simulink model "Ground_Vehicle_Model"  (R2020b)
settings: Solver=VariableStepAuto  StartTime=0.0  StopTime=40000  RelTol=1e-3
values from neighbouring files (symbols this model uses):
  waypoint = [waypoint(1,:);waypoint(1,:)]    [Path_Planning_Algorithm.m]
  Waypoint_Number = Waypoint_Number+1    [Path_Planning_Algorithm.m]
  waypoint_with_start = [0 0 0 0 0;waypoint]    [Path_Planning_Algorithm.m]
libraries: pid_lib x4, simulink x1, dspswit3 x1
settings Model: Creator=fuska  LastModifiedBy=fuska
settings DebuggingCC: AlgebraicLoopMsg=none

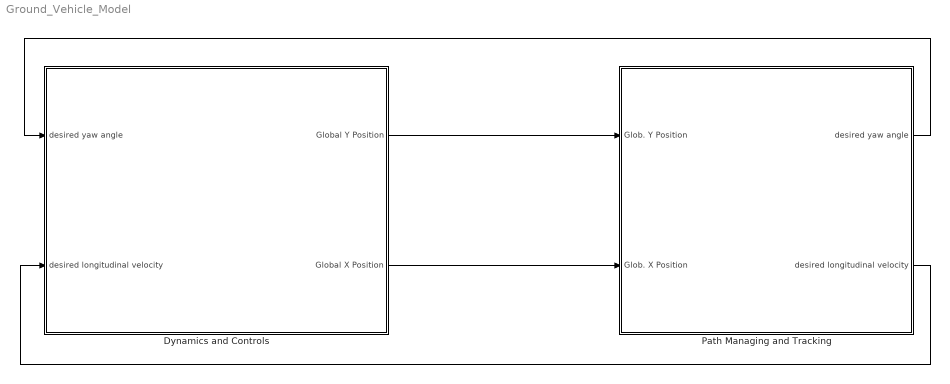
== system Ground_Vehicle_Model ==
  Dynamics and Controls : Subsystem
  Path Managing and Tracking : Subsystem
  wires:
  Dynamics and Controls/1(Global Y Position) -> Path Managing and Tracking/1(Glob. Y Position)
  Dynamics and Controls/2(Global X Position) -> Path Managing and Tracking/2(Glob. X Position)
  Path Managing and Tracking/1(desired yaw angle) -> Dynamics and Controls/1(desired yaw angle)
  Path Managing and Tracking/2(desired longitudinal velocity) -> Dynamics and Controls/2(desired longitudinal velocity)

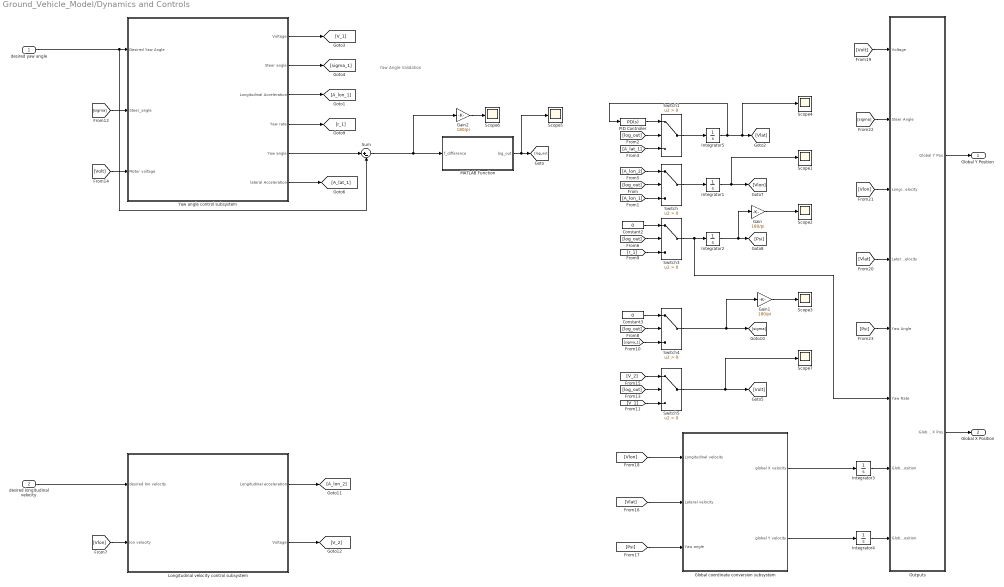
== system Ground_Vehicle_Model/Dynamics and Controls ==
  note: Yaw Angle Validation
  desired yaw angle : Inport
  desired longitudinal velocity : Inport  Port=2
  Constant2 : Constant  Value=0
  Constant3 : Constant  Value=0
  Gain : Gain  Gain=180/pi
  Gain1 : Gain  Gain=180/pi
  Gain2 : Gain  Gain=180/pi
  Global coordinate conversion subsystem : Subsystem
  Integrator{1..5} (5 alike) : Integrator
  Longitudinal velocity control subsystem : Subsystem
  MATLAB Function : MATLAB Function  TreatAsAtomicUnit=on
  Outputs : Subsystem
  PID Controller : pid_lib/PID Controller  Controller=PD  Form=Parallel  TimeDomain=Continuous-time  UseExternalTs=off  SampleTime=-1  IntegratorMethod=Forward Euler  FilterMethod=Forward Euler  ControllerParametersSource=internal  P=-0.8*9.81  I=1  D=0  UseFilter=on  N=100  TunerSelectOption=Transfer Function Based (PID Tuner App)  InitialConditionSource=internal  InitialConditionForIntegrator=0  InitialConditionForFilter=0  DifferentiatorICPrevScaledInput=0  ExternalReset=none  TrackingMode=off  Kt=1  LimitOutput=off  SatLimitsSource=internal  UpperSaturationLimit=inf  LowerSaturationLimit=-inf  LinearizeAsGain=on  AntiWindupMode=none  Kb=1  POutMin=[]  POutMax=[]  IOutMin=[]  IOutMax=[]  DOutMin=[]  DOutMax=[]  NOutMin=[]  NOutMax=[]  SumOutMin=[]  SumOutMax=[]  SaturationOutMin=[]  SaturationOutMax=[]  PParamMin=[]  PParamMax=[]  IParamMin=[]  IParamMax=[]  DParamMin=[]  DParamMax=[]  NParamMin=[]  NParamMax=[]  KbParamMin=[]  KbParamMax=[]  KtParamMin=[]  KtParamMax=[]  KbOutMin=[]  KbOutMax=[]  KtOutMin=[]  KtOutMax=[]  IntegratorOutMin=[]  IntegratorOutMax=[]  FilterOutMin=[]  FilterOutMax=[]  SumI1OutMin=[]  SumI1OutMax=[]  SumI2OutMin=[]  SumI2OutMax=[]  SumI3OutMin=[]  SumI3OutMax=[]  SumI4OutMin=[]  SumI4OutMax=[]  SumDOutMin=[]  SumDOutMax=[]  DifferentiatorOutMin=[]  DifferentiatorOutMax=[]  FilterDiffOutCoefMin=[]  FilterDiffOutCoefMax=[]  ReciprocalOutMin=[]  ReciprocalOutMax=[]  SumDenOutMin=[]  SumDenOutMax=[]  SumNumOutMin=[]  SumNumOutMax=[]  DivideOutMin=[]  DivideOutMax=[]  UdiffTsProdOutMin=[]  UdiffTsProdOutMax=[]  NTsProdOutMin=[]  NTsProdOutMax=[]  UintegralTsProdOutMin=[]  UintegralTsProdOutMax=[]  UngainTsProdOutMin=[]  UngainTsProdOutMax=[]  IntegratorContinuousStateAttributes=''  IntegratorStateMustResolveToSignalObject=off  IntegratorRTWStateStorageClass=Auto  FilterContinuousStateAttributes=''  FilterStateMustResolveToSignalObject=off  FilterRTWStateStorageClass=Auto  ParallelPVariant=InternalParameters  IdealPVariant=Disabled  IVariant=Disabled  DVariant=InternalParameters  IntegratorVariant=Disabled  SatVariant=Disabled  AWVariant=Disabled  PCopyVariant=Disabled  TRVariant=Disabled  FdbkBlocksVariant=Forward  IdealPFdbkVariant=Disabled  SatFdbkVariant=Disabled  DerivativeFilterVariant=ContFilter  NVariant=InternalParameters  NCopyVariant=Disabled  FilterICVariant=InternalICsFilter  IntegratorICVariant=Disabled  ExternalResetVariant=Disabled  TRSumVariant=Passthrough  SumFdbkVariant=Disabled  SumVariant=Sum_PD  TsampFilterVariant=InternalTs  TsampNgainVariant=Passthrough  TsampIntegralVariant=Disabled_SignalSpec  ExternalSaturationOutDataTypeStr=Inherit: Same as second input
  Scope{1..7} (7 alike) : Scope
  Sum : Sum  Inputs=|+-
  Switch{,1,3..5} (5 alike) : Switch  Criteria=u2 > Threshold
  Yaw angle control subsystem : Subsystem
  Global Y Position : Outport
  Global X Position : Outport  Port=2
  wires:
  desired yaw angle/1 -> Yaw angle control subsystem/1(Desired Yaw Angle), Sum/2
  Yaw angle control subsystem/5(Yaw angle) -> Sum/1
  Sum/1 -> Gain2/1, MATLAB Function/1(f_difference)
  MATLAB Function/1(log_out) -> Scope5/1, [log_out]
  [log_out] -> Switch/2
  Yaw angle control subsystem/3(Longitudinal Acceleration) -> [A_lon_1]
  [A_lon_1] -> Switch/3
  [A_lon_2] -> Switch/1
  Yaw angle control subsystem/1(Voltage) -> [V_1]
  Yaw angle control subsystem/2(Steer angle) -> [sigma_1]
  Switch/1 -> Integrator1/1
  Integrator1/1 -> Scope1/1, [Vlon]
  Integrator2/1 -> Gain/1, [Psi]
  Switch3/1 -> Outputs/6(Yaw Rate), Integrator2/1
  [log_out] -> Switch3/2
  [r_1] -> Switch3/3
  Constant2/1 -> Switch3/1
  Yaw angle control subsystem/4(Yaw rate) -> [r_1]
  Constant3/1 -> Switch4/1
  [sigma_1] -> Switch4/3
  [log_out] -> Switch4/2
  Switch4/1 -> Gain1/1, [sigma]
  [log_out] -> Switch5/2
  [V_1] -> Switch5/3
  Switch5/1 -> Scope7/1, [Volt]
  desired longitudinal velocity/1 -> Longitudinal velocity control subsystem/1(desired lon velocity)
  [Vlon] -> Longitudinal velocity control subsystem/2(lon velocity)
  Longitudinal velocity control subsystem/1(Longitudinal acceleration) -> [A_lon_2]
  Gain/1 -> Scope2/1
  [sigma] -> Yaw angle control subsystem/2(Steer_angle)
  Gain1/1 -> Scope3/1
  Gain2/1 -> Scope6/1
  [Volt] -> Yaw angle control subsystem/3(Motor voltage)
  Longitudinal velocity control subsystem/2(Voltage) -> [V_2]
  [V_2] -> Switch5/1
  Global coordinate conversion subsystem/1("global X velocity ") -> Integrator3/1
  [Vlon] -> Global coordinate conversion subsystem/1(Longitudinal velocity)
  [Vlat] -> Global coordinate conversion subsystem/2(Lateral velocity)
  Global coordinate conversion subsystem/2(global Y velocity) -> Integrator4/1
  [Psi] -> Global coordinate conversion subsystem/3(Yaw angle)
  [Volt] -> Outputs/1(Voltage)
  [Vlat] -> Outputs/4(Lateral Velocity)
  [Vlon] -> Outputs/3(Longitudinal Velocity)
  [sigma] -> Outputs/2(Steer Angle)
  [Psi] -> Outputs/5(Yaw Angle)
  Integrator3/1 -> Outputs/7(Global X Position)
  Integrator4/1 -> Outputs/8(Global Y Position)
  Switch1/1 -> Integrator5/1
  [log_out] -> Switch1/2
  [A_lat_1] -> Switch1/3
  Yaw angle control subsystem/6(lateral Acceleration) -> [A_lat_1]
  Integrator5/1 -> [Vlat], Scope4/1, PID Controller/1
  PID Controller/1 -> Switch1/1
  Outputs/2(Global X Pos.) -> Global X Position/1
  Outputs/1(Global Y Pos.) -> Global Y Position/1

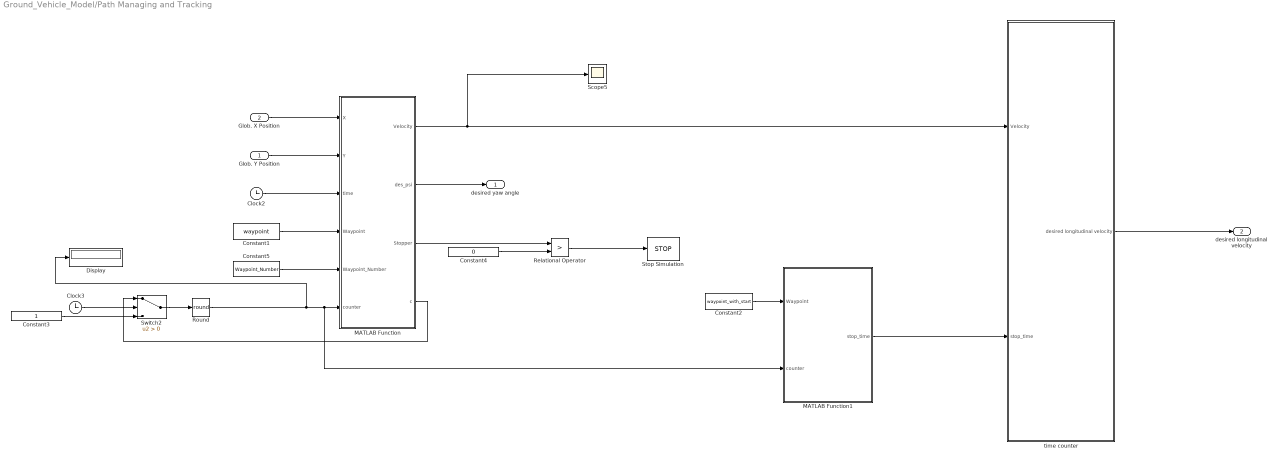
== system Ground_Vehicle_Model/Path Managing and Tracking ==
  Glob. Y Position : Inport
  Glob. X Position : Inport  Port=2
  Clock2 : Clock
  Clock3 : Clock
  Constant1 : Constant  Value=waypoint
  Constant2 : Constant  Value=waypoint_with_start
  Constant3 : Constant
  Constant4 : Constant  Value=0
  Constant5 : Constant  Value=Waypoint_Number
  Display : Display
  MATLAB Function : MATLAB Function  TreatAsAtomicUnit=on
  MATLAB Function1 : MATLAB Function  TreatAsAtomicUnit=on
  Relational Operator : RelationalOperator  Operator=>  OutDataTypeStr=boolean  RndMeth=Simplest
  Round : Rounding  Operator=round
  Scope5 : Scope
  Stop Simulation : Stop
  Switch2 : Switch  Criteria=u2 > Threshold  ZeroCross=off
  time counter : Subsystem
  desired yaw angle : Outport
  desired longitudinal velocity : Outport  Port=2
  wires:
  Glob. X Position/1 -> MATLAB Function/1(X)
  Clock2/1 -> MATLAB Function/3(time)
  Glob. Y Position/1 -> MATLAB Function/2(Y)
  Clock3/1 -> Switch2/2
  Constant3/1 -> Switch2/3
  Switch2/1 -> Round/1
  Round/1 -> MATLAB Function1/2(counter), MATLAB Function/6(counter), Display/1
  Relational Operator/1 -> Stop Simulation/1
  MATLAB Function/4(c) -> Switch2/1
  MATLAB Function/3(Stopper) -> Relational Operator/1
  Constant4/1 -> Relational Operator/2
  Constant5/1 -> MATLAB Function/5(Waypoint_Number)
  MATLAB Function/2(des_psi) -> desired yaw angle/1
  Constant2/1 -> MATLAB Function1/1(Waypoint)
  MATLAB Function/1(Velocity) -> Scope5/1, time counter/1(Velocity)
  time counter/1(desired longitudinal velocity) -> desired longitudinal velocity/1
  MATLAB Function1/1(stop_time) -> time counter/2(stop_time)
  Constant1/1 -> MATLAB Function/4(Waypoint)

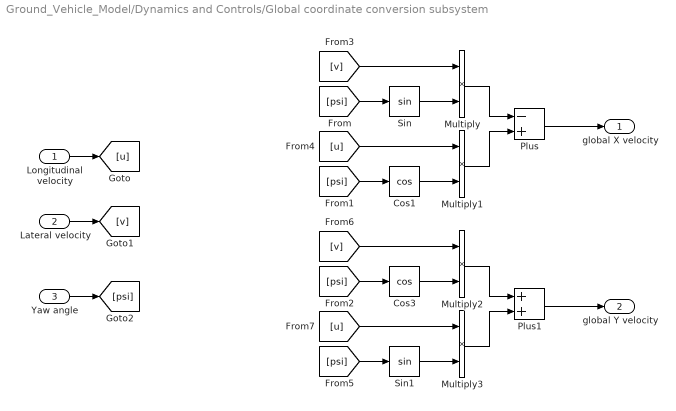
== system Ground_Vehicle_Model/Dynamics and Controls/Global coordinate conversion subsystem ==
  Longitudinal velocity : Inport
  Lateral velocity : Inport  Port=2
  Yaw angle : Inport  Port=3
  Cos1 : Trigonometry  Operator=cos
  Cos3 : Trigonometry  Operator=cos
  Multiply{,1..3} (4 alike) : Product
  Plus : Sum  Inputs=-+
  Plus1 : Sum
  Sin : Trigonometry
  Sin1 : Trigonometry
  "global X velocity " : Outport  VectorParamsAs1DForOutWhenUnconnected=off
  global Y velocity : Outport  Port=2  VectorParamsAs1DForOutWhenUnconnected=off
  wires:
  Longitudinal velocity/1 -> [u]
  Lateral velocity/1 -> [v]
  Yaw angle/1 -> [psi]
  [psi] -> Sin/1
  [psi] -> Cos1/1
  Sin/1 -> Multiply/2
  [v] -> Multiply/1
  [u] -> Multiply1/1
  Cos1/1 -> Multiply1/2
  Multiply/1 -> Plus/1
  Multiply1/1 -> Plus/2
  Multiply3/1 -> Plus1/2
  Multiply2/1 -> Plus1/1
  Sin1/1 -> Multiply3/2
  [u] -> Multiply3/1
  [v] -> Multiply2/1
  [psi] -> Sin1/1
  Plus1/1 -> global Y velocity/1
  Plus/1 -> "global X velocity "/1
  [psi] -> Cos3/1
  Cos3/1 -> Multiply2/2

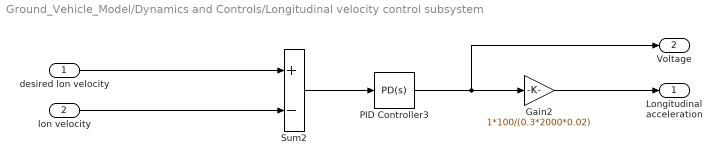
== system Ground_Vehicle_Model/Dynamics and Controls/Longitudinal velocity control subsystem ==
  desired lon velocity : Inport
  lon velocity : Inport  Port=2
  Gain2 : Gain  Gain=1*100/(0.3*2000*0.02)
  PID Controller3 : pid_lib/PID Controller  Controller=PD  Form=Parallel  TimeDomain=Continuous-time  UseExternalTs=off  SampleTime=-1  IntegratorMethod=Forward Euler  FilterMethod=Forward Euler  ControllerParametersSource=internal  P=1.23316781002483  I=235.883220320238  D=0.0859873397021034  UseFilter=on  N=17.2044274974478  TunerSelectOption=Transfer Function Based (PID Tuner App)  ZeroCross=off  InitialConditionSource=internal  InitialConditionForIntegrator=0  InitialConditionForFilter=0  DifferentiatorICPrevScaledInput=0  ExternalReset=none  TrackingMode=off  Kt=1  LimitOutput=on  SatLimitsSource=internal  UpperSaturationLimit=10  LowerSaturationLimit=-10  LinearizeAsGain=on  AntiWindupMode=none  Kb=1  POutMin=[]  POutMax=[]  IOutMin=[]  IOutMax=[]  DOutMin=[]  DOutMax=[]  NOutMin=[]  NOutMax=[]  SumOutMin=[]  SumOutMax=[]  SaturationOutMin=[]  SaturationOutMax=[]  PParamMin=[]  PParamMax=[]  IParamMin=[]  IParamMax=[]  DParamMin=[]  DParamMax=[]  NParamMin=[]  NParamMax=[]  KbParamMin=[]  KbParamMax=[]  KtParamMin=[]  KtParamMax=[]  KbOutMin=[]  KbOutMax=[]  KtOutMin=[]  KtOutMax=[]  IntegratorOutMin=[]  IntegratorOutMax=[]  FilterOutMin=[]  FilterOutMax=[]  SumI1OutMin=[]  SumI1OutMax=[]  SumI2OutMin=[]  SumI2OutMax=[]  SumI3OutMin=[]  SumI3OutMax=[]  SumI4OutMin=[]  SumI4OutMax=[]  SumDOutMin=[]  SumDOutMax=[]  DifferentiatorOutMin=[]  DifferentiatorOutMax=[]  FilterDiffOutCoefMin=[]  FilterDiffOutCoefMax=[]  ReciprocalOutMin=[]  ReciprocalOutMax=[]  SumDenOutMin=[]  SumDenOutMax=[]  SumNumOutMin=[]  SumNumOutMax=[]  DivideOutMin=[]  DivideOutMax=[]  UdiffTsProdOutMin=[]  UdiffTsProdOutMax=[]  NTsProdOutMin=[]  NTsProdOutMax=[]  UintegralTsProdOutMin=[]  UintegralTsProdOutMax=[]  UngainTsProdOutMin=[]  UngainTsProdOutMax=[]  IntegratorContinuousStateAttributes=''  IntegratorStateMustResolveToSignalObject=off  IntegratorRTWStateStorageClass=Auto  FilterContinuousStateAttributes=''  FilterStateMustResolveToSignalObject=off  FilterRTWStateStorageClass=Auto  ParallelPVariant=InternalParameters  IdealPVariant=Disabled  IVariant=Disabled  DVariant=InternalParameters  IntegratorVariant=Disabled  SatVariant=Enabled  AWVariant=Disabled  PCopyVariant=Disabled  TRVariant=Disabled  FdbkBlocksVariant=Forward  IdealPFdbkVariant=Disabled  SatFdbkVariant=Disabled  DerivativeFilterVariant=ContFilter  NVariant=InternalParameters  NCopyVariant=Disabled  FilterICVariant=InternalICsFilter  IntegratorICVariant=Disabled  ExternalResetVariant=Disabled  TRSumVariant=Passthrough  SumFdbkVariant=Disabled  SumVariant=Sum_PD  TsampFilterVariant=InternalTs  TsampNgainVariant=Passthrough  TsampIntegralVariant=Disabled_SignalSpec  ExternalSaturationOutDataTypeStr=Inherit: Same as second input
  Sum2 : Sum  Inputs=+-
  Longitudinal acceleration : Outport
  Voltage : Outport  Port=2
  wires:
  Sum2/1 -> PID Controller3/1
  Gain2/1 -> Longitudinal acceleration/1
  PID Controller3/1 -> Voltage/1, Gain2/1
  desired lon velocity/1 -> Sum2/1
  lon velocity/1 -> Sum2/2

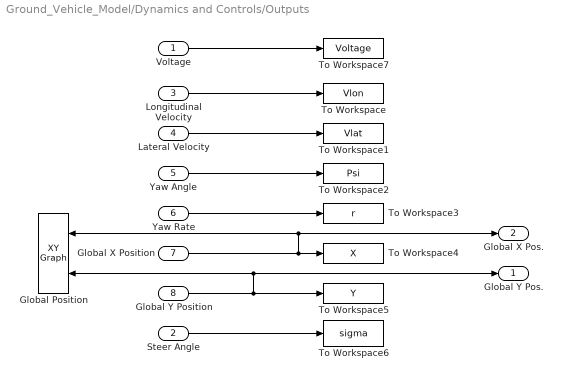
== system Ground_Vehicle_Model/Dynamics and Controls/Outputs ==
  Voltage : Inport
  Steer Angle : Inport  Port=2
  Longitudinal Velocity : Inport  Port=3
  Lateral Velocity : Inport  Port=4
  Yaw Angle : Inport  Port=5
  Yaw Rate : Inport  Port=6
  Global X Position : Inport  Port=7
  Global Y Position : Inport  Port=8
  "Global Position " : simulink/Sinks/XY Graph  xmin=-inf  xmax=inf  ymin=-inf  ymax=inf  st=-1
  To Workspace : ToWorkspace  VariableName=Vlon  SaveFormat=Timeseries  SampleTime=-1
  To Workspace1 : ToWorkspace  VariableName=Vlat  SaveFormat=Timeseries  SampleTime=-1
  To Workspace2 : ToWorkspace  VariableName=Psi  SaveFormat=Timeseries  SampleTime=-1
  To Workspace3 : ToWorkspace  VariableName=r  SaveFormat=Timeseries  SampleTime=-1
  To Workspace4 : ToWorkspace  VariableName=X  SaveFormat=Timeseries  SampleTime=-1
  To Workspace5 : ToWorkspace  VariableName=Y  SaveFormat=Timeseries  SampleTime=-1
  To Workspace6 : ToWorkspace  VariableName=sigma  SaveFormat=Timeseries  SampleTime=-1
  To Workspace7 : ToWorkspace  VariableName=Voltage  SaveFormat=Timeseries  SampleTime=-1
  Global Y Pos. : Outport
  Global X Pos. : Outport  Port=2
  wires:
  Yaw Rate/1 -> To Workspace3/1
  Yaw Angle/1 -> To Workspace2/1
  Global X Position/1 -> Global X Pos./1, "Global Position "/1, To Workspace4/1
  Lateral Velocity/1 -> To Workspace1/1
  Longitudinal Velocity/1 -> To Workspace/1
  Voltage/1 -> To Workspace7/1
  Steer Angle/1 -> To Workspace6/1
  Global Y Position/1 -> To Workspace5/1, Global Y Pos./1, "Global Position "/2

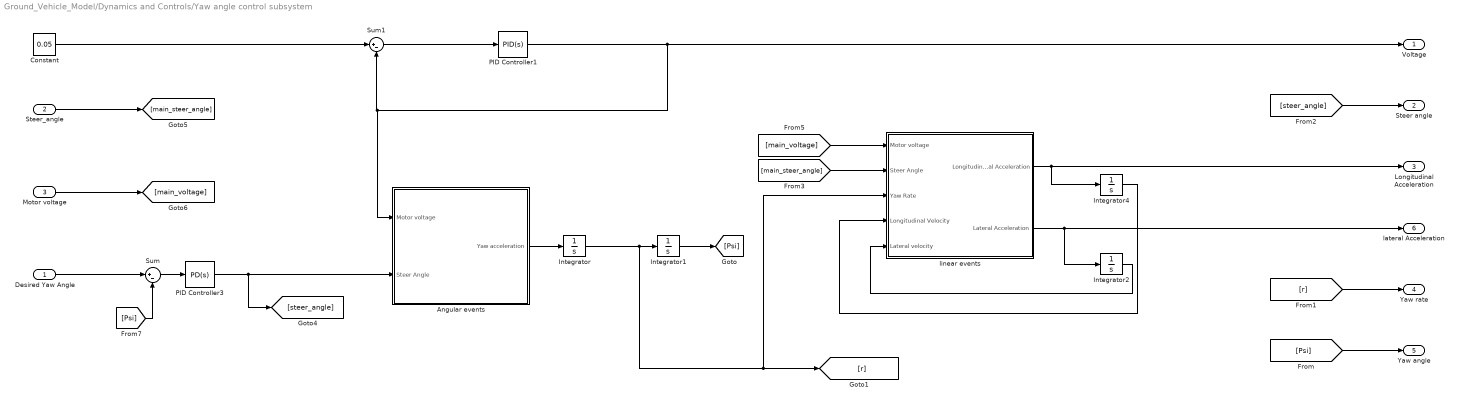
== system Ground_Vehicle_Model/Dynamics and Controls/Yaw angle control subsystem ==
  Desired Yaw Angle : Inport
  Steer_angle : Inport  Port=2
  Motor voltage : Inport  Port=3
  Angular events : Subsystem
  Constant : Constant  Value=0.05
  Integrator{,1..2,4} (4 alike) : Integrator
  PID Controller1 : pid_lib/PID Controller  Controller=PID  Form=Parallel  TimeDomain=Continuous-time  UseExternalTs=off  SampleTime=-1  IntegratorMethod=Forward Euler  FilterMethod=Forward Euler  ControllerParametersSource=internal  P=0  I=1  D=0  UseFilter=on  N=100  TunerSelectOption=Transfer Function Based (PID Tuner App)  InitialConditionSource=internal  InitialConditionForIntegrator=0  InitialConditionForFilter=0  DifferentiatorICPrevScaledInput=0  ExternalReset=none  TrackingMode=off  Kt=1  LimitOutput=off  SatLimitsSource=internal  UpperSaturationLimit=inf  LowerSaturationLimit=-inf  LinearizeAsGain=on  AntiWindupMode=none  Kb=1  POutMin=[]  POutMax=[]  IOutMin=[]  IOutMax=[]  DOutMin=[]  DOutMax=[]  NOutMin=[]  NOutMax=[]  SumOutMin=[]  SumOutMax=[]  SaturationOutMin=[]  SaturationOutMax=[]  PParamMin=[]  PParamMax=[]  IParamMin=[]  IParamMax=[]  DParamMin=[]  DParamMax=[]  NParamMin=[]  NParamMax=[]  KbParamMin=[]  KbParamMax=[]  KtParamMin=[]  KtParamMax=[]  KbOutMin=[]  KbOutMax=[]  KtOutMin=[]  KtOutMax=[]  IntegratorOutMin=[]  IntegratorOutMax=[]  FilterOutMin=[]  FilterOutMax=[]  SumI1OutMin=[]  SumI1OutMax=[]  SumI2OutMin=[]  SumI2OutMax=[]  SumI3OutMin=[]  SumI3OutMax=[]  SumI4OutMin=[]  SumI4OutMax=[]  SumDOutMin=[]  SumDOutMax=[]  DifferentiatorOutMin=[]  DifferentiatorOutMax=[]  FilterDiffOutCoefMin=[]  FilterDiffOutCoefMax=[]  ReciprocalOutMin=[]  ReciprocalOutMax=[]  SumDenOutMin=[]  SumDenOutMax=[]  SumNumOutMin=[]  SumNumOutMax=[]  DivideOutMin=[]  DivideOutMax=[]  UdiffTsProdOutMin=[]  UdiffTsProdOutMax=[]  NTsProdOutMin=[]  NTsProdOutMax=[]  UintegralTsProdOutMin=[]  UintegralTsProdOutMax=[]  UngainTsProdOutMin=[]  UngainTsProdOutMax=[]  IntegratorContinuousStateAttributes=''  IntegratorStateMustResolveToSignalObject=off  IntegratorRTWStateStorageClass=Auto  FilterContinuousStateAttributes=''  FilterStateMustResolveToSignalObject=off  FilterRTWStateStorageClass=Auto  ParallelPVariant=InternalParameters  IdealPVariant=Disabled  IVariant=InternalParameters  DVariant=InternalParameters  IntegratorVariant=Continuous  SatVariant=Disabled  AWVariant=Passthrough  PCopyVariant=Disabled  TRVariant=Disabled  FdbkBlocksVariant=Forward  IdealPFdbkVariant=Disabled  SatFdbkVariant=Disabled  DerivativeFilterVariant=ContFilter  NVariant=InternalParameters  NCopyVariant=Disabled  FilterICVariant=InternalICsFilter  IntegratorICVariant=InternalICs  ExternalResetVariant=Disabled  TRSumVariant=Passthrough  SumFdbkVariant=Disabled  SumVariant=Sum_PID  TsampFilterVariant=InternalTs  TsampNgainVariant=Passthrough  TsampIntegralVariant=Passthrough  ExternalSaturationOutDataTypeStr=Inherit: Same as second input
  PID Controller3 : pid_lib/PID Controller  Controller=PD  Form=Parallel  TimeDomain=Continuous-time  UseExternalTs=off  SampleTime=-1  IntegratorMethod=Forward Euler  FilterMethod=Forward Euler  ControllerParametersSource=internal  P=1.84296120420569  I=93.7992974389489  D=3.62409743962699  UseFilter=on  N=54.8881885391225  TunerSelectOption=Transfer Function Based (PID Tuner App)  ZeroCross=off  InitialConditionSource=internal  InitialConditionForIntegrator=0  InitialConditionForFilter=0  DifferentiatorICPrevScaledInput=0  ExternalReset=none  TrackingMode=off  Kt=1  LimitOutput=on  SatLimitsSource=internal  UpperSaturationLimit=60*pi/180  LowerSaturationLimit=-60*pi/180  LinearizeAsGain=off  AntiWindupMode=none  Kb=1  POutMin=[]  POutMax=[]  IOutMin=[]  IOutMax=[]  DOutMin=[]  DOutMax=[]  NOutMin=[]  NOutMax=[]  SumOutMin=[]  SumOutMax=[]  SaturationOutMin=[]  SaturationOutMax=[]  PParamMin=[]  PParamMax=[]  IParamMin=[]  IParamMax=[]  DParamMin=[]  DParamMax=[]  NParamMin=[]  NParamMax=[]  KbParamMin=[]  KbParamMax=[]  KtParamMin=[]  KtParamMax=[]  KbOutMin=[]  KbOutMax=[]  KtOutMin=[]  KtOutMax=[]  IntegratorOutMin=[]  IntegratorOutMax=[]  FilterOutMin=[]  FilterOutMax=[]  SumI1OutMin=[]  SumI1OutMax=[]  SumI2OutMin=[]  SumI2OutMax=[]  SumI3OutMin=[]  SumI3OutMax=[]  SumI4OutMin=[]  SumI4OutMax=[]  SumDOutMin=[]  SumDOutMax=[]  DifferentiatorOutMin=[]  DifferentiatorOutMax=[]  FilterDiffOutCoefMin=[]  FilterDiffOutCoefMax=[]  ReciprocalOutMin=[]  ReciprocalOutMax=[]  SumDenOutMin=[]  SumDenOutMax=[]  SumNumOutMin=[]  SumNumOutMax=[]  DivideOutMin=[]  DivideOutMax=[]  UdiffTsProdOutMin=[]  UdiffTsProdOutMax=[]  NTsProdOutMin=[]  NTsProdOutMax=[]  UintegralTsProdOutMin=[]  UintegralTsProdOutMax=[]  UngainTsProdOutMin=[]  UngainTsProdOutMax=[]  IntegratorContinuousStateAttributes=''  IntegratorStateMustResolveToSignalObject=off  IntegratorRTWStateStorageClass=Auto  FilterContinuousStateAttributes=''  FilterStateMustResolveToSignalObject=off  FilterRTWStateStorageClass=Auto  ParallelPVariant=InternalParameters  IdealPVariant=Disabled  IVariant=Disabled  DVariant=InternalParameters  IntegratorVariant=Disabled  SatVariant=Enabled  AWVariant=Disabled  PCopyVariant=Disabled  TRVariant=Disabled  FdbkBlocksVariant=Forward  IdealPFdbkVariant=Disabled  SatFdbkVariant=Disabled  DerivativeFilterVariant=ContFilter  NVariant=InternalParameters  NCopyVariant=Disabled  FilterICVariant=InternalICsFilter  IntegratorICVariant=Disabled  ExternalResetVariant=Disabled  TRSumVariant=Passthrough  SumFdbkVariant=Disabled  SumVariant=Sum_PD  TsampFilterVariant=InternalTs  TsampNgainVariant=Passthrough  TsampIntegralVariant=Disabled_SignalSpec  ExternalSaturationOutDataTypeStr=Inherit: Same as second input
  Sum : Sum  Inputs=|+-
  Sum1 : Sum  Inputs=|+-
  linear events : Subsystem
  Voltage : Outport
  Steer angle : Outport  Port=2
  Longitudinal Acceleration : Outport  Port=3
  Yaw rate : Outport  Port=4
  Yaw angle : Outport  Port=5
  lateral Acceleration : Outport  Port=6
  wires:
  linear events/1(Longitudinal Acceleration) -> Integrator4/1, Longitudinal Acceleration/1
  Sum/1 -> PID Controller3/1
  Desired Yaw Angle/1 -> Sum/1
  Integrator4/1 -> linear events/4(Longitudinal Velocity)
  Sum1/1 -> PID Controller1/1
  Constant/1 -> Sum1/1
  [Psi] -> Yaw angle/1
  [r] -> Yaw rate/1
  Steer_angle/1 -> [main_steer_angle]
  [steer_angle] -> Steer angle/1
  [main_steer_angle] -> linear events/2(Steer Angle)
  Motor voltage/1 -> [main_voltage]
  [main_voltage] -> linear events/1(Motor voltage)
  PID Controller1/1 -> Voltage/1, Angular events/1(Motor voltage), Sum1/2
  PID Controller3/1 -> Angular events/2(Steer Angle), [steer_angle]
  Angular events/1(Yaw acceleration) -> Integrator/1
  Integrator1/1 -> [Psi]
  Integrator/1 -> linear events/3(Yaw Rate), [r], Integrator1/1
  [Psi] -> Sum/2
  linear events/2(Lateral Acceleration) -> Integrator2/1, lateral Acceleration/1
  Integrator2/1 -> linear events/5(Lateral velocity)

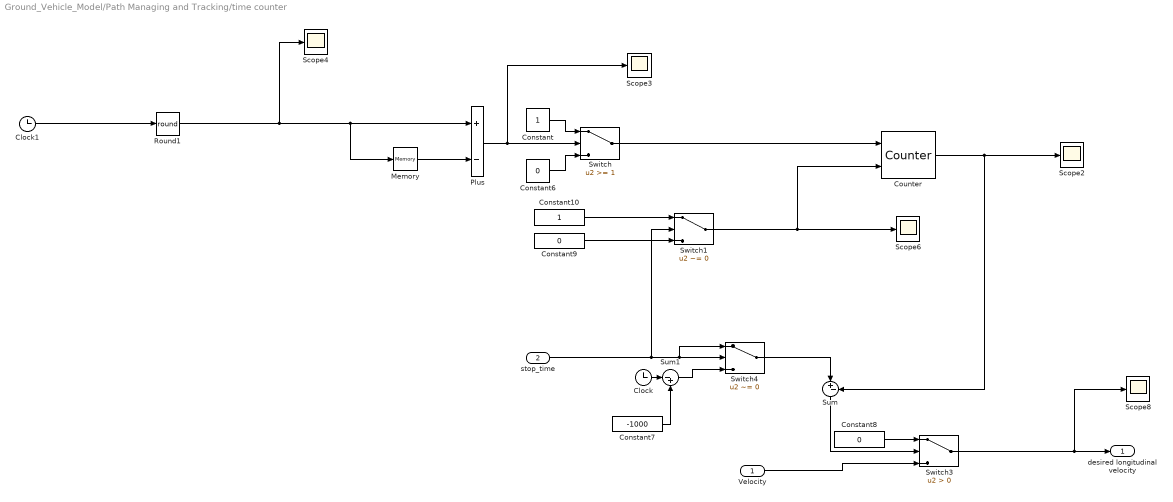
== system Ground_Vehicle_Model/Path Managing and Tracking/time counter ==
  Velocity : Inport
  stop_time : Inport  Port=2
  Clock : Clock
  Clock1 : Clock
  Constant : Constant
  Constant10 : Constant
  Constant6 : Constant  Value=0
  Constant7 : Constant  Value=-1000
  Constant8 : Constant  Value=0
  Constant9 : Constant  Value=0
  Counter : dspswit3/Counter  Direction=Up  CountEvent=Rising edge  CounterSize=User defined  MaxCount=500  InitialCount=0  Output=Count  HitValue=32  ResetInput=on  SamplesPerFrame=1  Ts=1  CntDtype=double  HitDtype=Logical
  Memory : Memory
  Plus : Sum  Inputs=+-
  Round1 : Rounding  Operator=round
  Scope{2..4,6,8} (5 alike) : Scope
  Sum : Sum  Inputs=|+-
  Sum1 : Sum  Inputs=|-+
  Switch : Switch  Threshold=1
  Switch1 : Switch  Criteria=u2 ~= 0  Threshold=1
  Switch3 : Switch  Criteria=u2 > Threshold
  Switch4 : Switch  Criteria=u2 ~= 0  Threshold=1
  desired longitudinal velocity : Outport
  wires:
  Memory/1 -> Plus/2
  Plus/1 -> Scope3/1, Switch/2
  Round1/1 -> Scope4/1, Memory/1, Plus/1
  Constant10/1 -> Switch1/1
  Constant6/1 -> Switch/3
  Counter/1 -> Sum/2, Scope2/1
  Switch/1 -> Counter/1
  Constant/1 -> Switch/1
  Switch3/1 -> Scope8/1, desired longitudinal velocity/1
  Constant7/1 -> Sum1/2
  Clock/1 -> Sum1/1
  Clock1/1 -> Round1/1
  Switch4/1 -> Sum/1
  Sum1/1 -> Switch4/3
  Switch1/1 -> Scope6/1, Counter/2
  Constant9/1 -> Switch1/3
  Sum/1 -> Switch3/2
  Constant8/1 -> Switch3/1
  Velocity/1 -> Switch3/3
  stop_time/1 -> Switch1/2, Switch4/1, Switch4/2

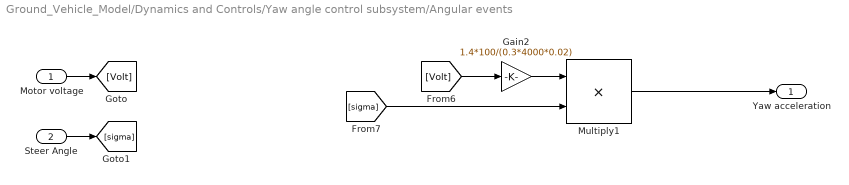
== system Ground_Vehicle_Model/Dynamics and Controls/Yaw angle control subsystem/Angular events ==
  Motor voltage : Inport
  Steer Angle : Inport  Port=2
  Gain2 : Gain  Gain=1.4*100/(0.3*4000*0.02)
  Multiply1 : Product
  Yaw acceleration : Outport
  wires:
  Multiply1/1 -> Yaw acceleration/1
  [Volt] -> Gain2/1
  [sigma] -> Multiply1/2
  Motor voltage/1 -> [Volt]
  Steer Angle/1 -> [sigma]
  Gain2/1 -> Multiply1/1

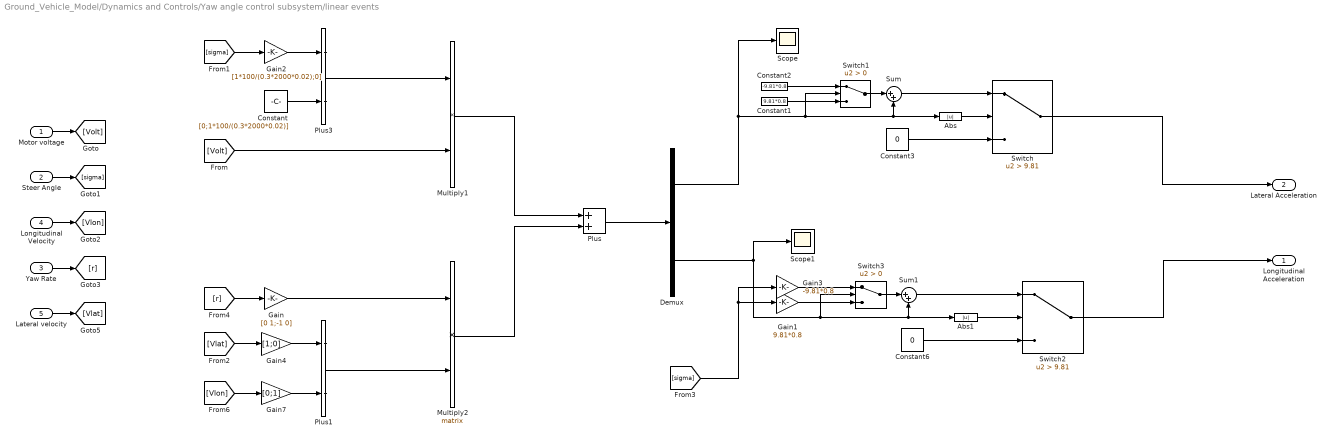
== system Ground_Vehicle_Model/Dynamics and Controls/Yaw angle control subsystem/linear events ==
  Motor voltage : Inport
  Steer Angle : Inport  Port=2
  Yaw Rate : Inport  Port=3
  Longitudinal Velocity : Inport  Port=4
  Lateral velocity : Inport  Port=5
  Abs : Abs
  Abs1 : Abs
  Constant : Constant  Value=[0;1*100/(0.3*2000*0.02)]
  Constant1 : Constant  Value=9.81*0.8
  Constant2 : Constant  Value=-9.81*0.8
  Constant3 : Constant  Value=0
  Constant6 : Constant  Value=0
  Demux : Demux  Outputs=2
  Gain : Gain  Gain=[0 1;-1 0]
  Gain1 : Gain  Gain=9.81*0.8
  Gain2 : Gain  Gain=[1*100/(0.3*2000*0.02);0]
  Gain3 : Gain  Gain=-9.81*0.8
  Gain4 : Gain  Gain=[1;0]
  Gain7 : Gain  Gain=[0;1]
  Multiply1 : Product
  Multiply2 : Product  Multiplication=Matrix(*)
  Plus : Sum
  Plus1 : Sum
  Plus3 : Sum
  Scope : Scope
  Scope1 : Scope
  Sum : Sum  Inputs=|++
  Sum1 : Sum  Inputs=|++
  Switch : Switch  Criteria=u2 > Threshold  Threshold=9.81
  Switch1 : Switch  Criteria=u2 > Threshold
  Switch2 : Switch  Criteria=u2 > Threshold  Threshold=9.81
  Switch3 : Switch  Criteria=u2 > Threshold
  Longitudinal Acceleration : Outport  VectorParamsAs1DForOutWhenUnconnected=off
  Lateral Acceleration : Outport  Port=2  VectorParamsAs1DForOutWhenUnconnected=off
  wires:
  Motor voltage/1 -> [Volt]
  Steer Angle/1 -> [sigma]
  Yaw Rate/1 -> [r]
  Longitudinal Velocity/1 -> [Vlon]
  Lateral velocity/1 -> [Vlat]
  Gain4/1 -> Plus1/1
  [Volt] -> Multiply1/2
  Gain/1 -> Multiply2/1
  Plus/1 -> Demux/1
  Plus3/1 -> Multiply1/1
  Gain2/1 -> Plus3/1
  Constant/1 -> Plus3/2
  [Vlat] -> Gain4/1
  [sigma] -> Gain2/1
  [Vlon] -> Gain7/1
  Gain7/1 -> Plus1/2
  Multiply1/1 -> Plus/1
  Plus1/1 -> Multiply2/2
  Multiply2/1 -> Plus/2
  [r] -> Gain/1
  Demux/1 -> Scope/1, Switch1/2, Sum/2, Abs/1
  Sum/1 -> Switch/1
  Abs/1 -> Switch/2
  Switch1/1 -> Sum/1
  Constant2/1 -> Switch1/1
  Constant1/1 -> Switch1/3
  Constant3/1 -> Switch/3
  Switch/1 -> Lateral Acceleration/1
  Gain3/1 -> Switch3/1
  Gain1/1 -> Switch3/3
  Abs1/1 -> Switch2/2
  Constant6/1 -> Switch2/3
  Demux/2 -> Switch3/2, Sum1/2, Abs1/1, Scope1/1
  Switch3/1 -> Sum1/1
  Sum1/1 -> Switch2/1
  Switch2/1 -> Longitudinal Acceleration/1
  [sigma] -> Gain3/1, Gain1/1

== matlab function Ground_Vehicle_Model/Path Managing and Tracking/MATLAB Function ==
  data: Velocity output; des_psi output; Stopper output; X input; Y input; time input; c output; Waypoint input; Waypoint_Number input; counter input
function [Velocity,des_psi,Stopper,c] = fcn(X,Y,time,Waypoint,Waypoint_Number,counter)
if time==0 || counter==0;
a=1;
else 
    a=counter;
end
X_target=Waypoint(a,1);
Y_target=Waypoint(a,2);
Velocity=Waypoint(a,3);
turn=Waypoint(a,5);
dist_y=Y_target-Y;
dist_x=X_target-X;
des_psi=atan2(dist_y,dist_x);

if abs(turn)>0
  if des_psi>turn+abs(285.007*(pi/180)^2/turn)
    des_psi=des_psi-360*pi/180; 
    end
end

dist=sqrt(dist_y^2+dist_x^2);
if dist<1
  c=counter+1;
else
    c=counter;
end

if c>Waypoint_Number
    c=c-1;
    Stopper=1;
else
    Stopper=0;
end
end

== matlab function Ground_Vehicle_Model/Dynamics and Controls/MATLAB Function ==
  data: f_difference input; log_out output
function log_out = fcn(f_difference)
if abs(f_difference)<(0.001*pi/180)
    log_out=1;
else
    log_out=0;
end
end

== matlab function Ground_Vehicle_Model/Path Managing and Tracking/MATLAB Function1 ==
  data: Waypoint input; counter input; stop_time output
function stop_time  = fcn(Waypoint,counter)
stop_time=Waypoint(counter,4);
end
